simulink model "izhikevich"  (R2020a)
settings: Solver=VariableStepAuto  StartTime=0.0  StopTime=STOP  RelTol=1e-3
values from neighbouring files (symbols this model uses):
  a = param(1)    [params.m]
  b = param(2)    [params.m]
  c = param(3)    [params.m]
  d = param(4)    [params.m]
  I = param(5)    [params.m]
  STOP = 500    [params.m]
settings Model: Creator=40175607  LastModifiedBy=40175607

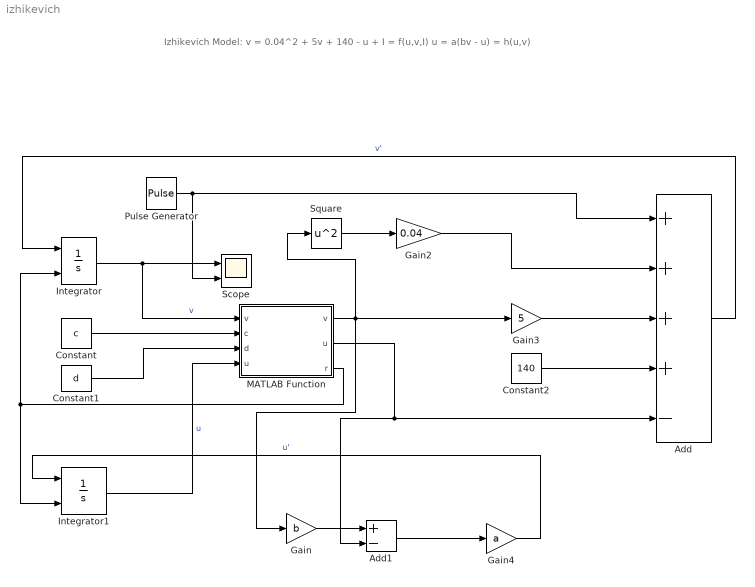
== system izhikevich ==
  note: Izhikevich Model:
      |
      | v = 0.04^2 + 5v + 140 - u + I = f(u,v,I)
      | u = a(bv - u) = h(u,v)
  Add : Sum  Inputs=++++-
  Add1 : Sum  Inputs=+-
  Constant : Constant  Value=c
  Constant1 : Constant  Value=d
  Constant2 : Constant  Value=140
  Gain : Gain  Gain=b
  Gain2 : Gain  Gain=0.04
  Gain3 : Gain  Gain=5
  Gain4 : Gain  Gain=a
  Integrator : Integrator  ExternalReset=rising  InitialCondition=c  LimitOutput=on  UpperSaturationLimit=30
  Integrator1 : Integrator  ExternalReset=rising  InitialCondition=d  LimitOutput=on
  MATLAB Function : MATLAB Function  TreatAsAtomicUnit=on
  Pulse Generator : DiscretePulseGenerator  PulseType=Time based  Amplitude=I  Period=STOP/2  PulseWidth=50  PhaseDelay=40
  Scope : Scope  NumInputPorts=2
  Square : Math  Operator=square  SaturateOnIntegerOverflow=on
  wires:
  Integrator1/1 -> MATLAB Function/4("u ")  "u"
  Integrator/1 -> MATLAB Function/1("v "), Scope/1  "v"
  Add/1 -> Integrator/1  "v'"
  Gain4/1 -> Integrator1/1  "u'"
  Square/1 -> Gain2/1
  Pulse Generator/1 -> Add/1, Scope/2
  Gain2/1 -> Add/2
  Gain3/1 -> Add/3
  Constant2/1 -> Add/4
  Add1/1 -> Gain4/1
  Gain/1 -> Add1/1
  Constant/1 -> MATLAB Function/2(c)
  Constant1/1 -> MATLAB Function/3(d)
  MATLAB Function/1(v) -> Gain/1, Square/1, Gain3/1
  MATLAB Function/2(u) -> Add/5, Add1/2
  MATLAB Function/3(r) -> Integrator/2, Integrator1/2

== matlab function izhikevich/MATLAB Function ==
  data: v input; c input; d input; u input; v output; u output; r output
function [v,u,r] = fcn(v,c,d,u)

if v>= 30
    v = c;
    u = c+d;
    r = 1;
else
    r=0;
end

y = u;
